simulink model "RF_FFT_Ex1"  (R2025a)
settings: Solver=ode45  StopTime=1024/10e3  EnableMultiTasking=on
InitFcn:
  | FFT_Size = 64;
undefined symbols (not defined in the file): i, S, vsva2488, xcvr1602
libraries: hdlBasic x15, dspsrcs4 x1, hdlDSPIP x1, dspxfrm3 x1, vmcUtilities x1
settings Model: Creator=dahlawat  LastModifiedBy=robg
settings SolverCC: AlgebraicLoopSolver=TrustRegion
settings DataIOCC: LimitDataPoints=on  SaveFormat=Array  ReturnWorkspaceOutputs=off
settings OptimizationCC: LifeSpan=inf
settings DebuggingCC: SolverPrmCheckMsg=warning  UnconnectedInputMsg=warning  UnconnectedOutputMsg=warning  UnconnectedLineMsg=warning  StateNameClashWarn=warning  SFUnexpectedBacktrackingDiag=warning  SFNoUnconditionalDefaultTransitionDiag=warning  SFExecutionAtInitializationDiag=none  ArithmeticOperatorsInVariantConditions=warning
settings HardwareCC: ProdBitPerPointer=32.0  ProdBitPerSizeT=32.0  ProdBitPerPtrDiffT=32.0  ProdLargestAtomicFloat=None  ProdIntDivRoundTo=Undefined  ProdEndianess=Unspecified  ProdWordSize=32.0  ProdHWDeviceType=32-bit Generic
settings ModelReferenceCC: EnableRefExpFcnMdlSchedulingChecks=on
settings SFSimCC: SimUseLocalCustomCode=off  CustomCodeUndefinedFunction=UseInterfaceOnly
settings RTWCC: RTWUseLocalCustomCode=off  GPUComputeCapability=3.5  DLArmComputeVersion=19.05
settings CodeAppCC: StateflowObjectComments=on
settings GRTTargetCC: TargetLangStandard=C89/C90 (ANSI)
settings ConfigComp: CovMetricSettings=dw  CovSaveCumulativeToWorkspaceVar=on  CovSaveSingleToWorkspaceVar=on  CovExternalEMLEnable=off

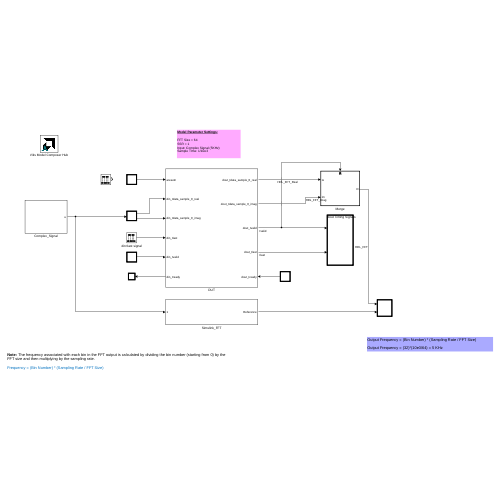
[thumbnail: Simulink's stored preview of the top-level diagram]
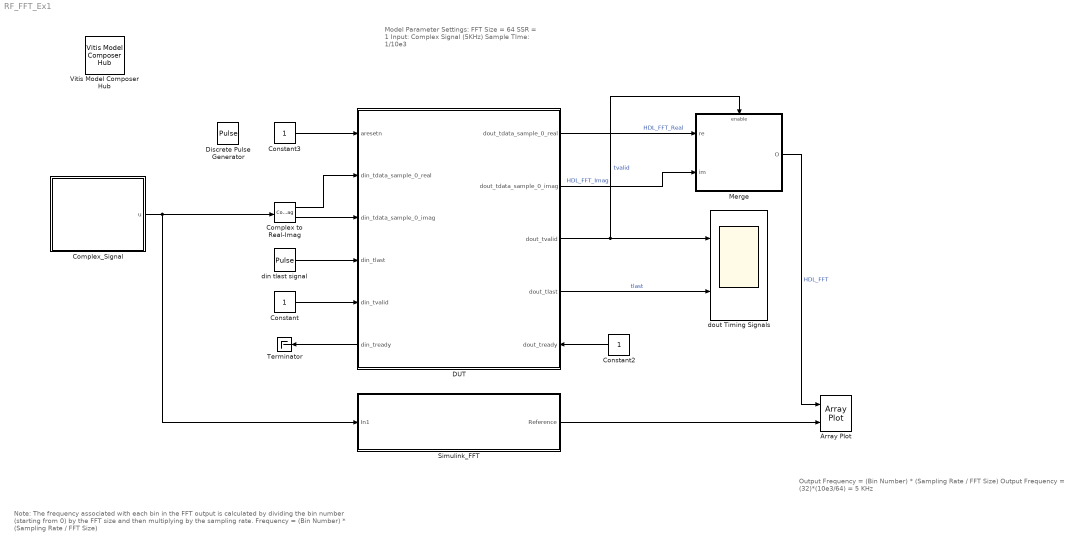
== system RF_FFT_Ex1 ==
  note: Output Frequency = (Bin Number) * (Sampling Rate / FFT Size)
      |
      | Output Frequency = (32)*(10e3/64) = 5 KHz
  note: Note: The frequency associated with each bin in the FFT output is calculated by dividing the bin number (starting from 0) by the FFT size and then multiplying by the sampling rate.
      |
      | Frequency = (Bin Number) * (Sampling Rate / FFT Size)
  note: Model Parameter Settings:
      |
      | FFT Size = 64
      | SSR = 1
      | Input: Complex Signal (5KHz)
      | Sample TIme: 1/10e3
  Array Plot : ArrayPlot  NumInputPorts=2  WindowPosition=[6.000000,33.000000,1920.000000,1149.000000,]  Visible=on  ScopeFrameLocation=window  YLimits=[-0.0625 0.5625]  ShowLegend=on
  Complex to Real-Imag : ComplexToRealImag
  Complex_Signal : Subsystem
  Constant : Constant
  Constant2 : Constant
  Constant3 : Constant
  DUT : Subsystem
      settings: PortSchema="{\"entries\":[{\"content\":{\"sides\":[{\"content\":{\"connectorIds\":[\"In1\",\"In2\",\"In3\",\"In4\",\"In5\",\"Out5\"]},\"type\":\"ConnectorPlacement.EquallySpacedRectSide\",\"uuid\":\"3c6f3837-184a-448e-85f8-bb0a441efaec\"},{\"content\":{\"connectorIds\":[\"Out1\",\"Out2\",\"Out3\",\"Out4\",\"In6\"],\"side\":\"RIGHT\"},\"type\":\"ConnectorPlacement.EquallySpacedRectSide\",\"uuid\":\"46fc4b89-da5b-4d62-9143-13f654c886da\"},{\"content\":{\"side\":\"TOP\"},\"type\":\"ConnectorPlacement.EquallySpacedRectSide\",\"uuid\":\"2ecc5b63-43c6-41c4-888c-4e2ddc41af1e\"}]},\"type\":\"ConnectorPlacement.EquallySpacedConnector\",\"uuid\":\"ba77804d-286f-47a8-b8da-0557eabd74b9\"}],\"packageUris\":[\"http://schema.mathworks.com/mf0/Connector/R2020b\"],\"version\":\"1.0\"}"
  Discrete Pulse Generator : DiscretePulseGenerator  Period=1  SampleTime=1/1e4
  Merge : Subsystem
  Simulink_FFT : Subsystem
  Terminator : Terminator
  Vitis Model Composer Hub : vmcUtilities/Vitis Model Composer Hub  Tag=genX  CodeGeneration=off  SubsystemName=DUT  CompilationType=HDLCompilation  SubsystemType=HDLNode  ExportTypeV2=IP Catalog  StartColumn=1  NumberOfColumns=1  TargetDirectory=./netlist  exportDesign=off  analyzeDesign=on  validateDesignOnHw=off  ExportType=HW Code  IpVendor=xilinx.com  IpLibrary=hls  IpVersion=1.0  IpHWLanguage=Verilog  AieCompilerOptions={}  AieSimulatorOptions={}  CreateTestbench=on  TestbenchStackSize=10  RunRtlSim=off  RunCSim=off  RunAieSim=on  enableSimulationTimeout=on  enableGraphIterations=on  AieSimTimeout=50000  AieGraphIterations=-1  RunAieSimProfiling=off  LaunchVitisAnalyzer=off  PlotOutput=off  RunX86Sim=off  X86SimTimeout=10  GenHwImage=off  GenLibadfXo=on  GenHwValidationCode=off  PlatformType=Not Specified  HwSystemType=Baremetal  HwValidationTarget=hw  ProjDevice=xcvr1602-vsva2488-2HP-i-S  ProjDevicePart=xcvr1602-vsva2488-2HP-i-S  AIEType=AIE  SamplePeriod=-1  ClockFrequency=200  DataPathParallelism=1  xilinxfamily=versalrf  part=xcvr1602  speed=-2HP-i-S  package=vsva2488  directory=./netlist/ip/DUT/src  testbench=off  incr_netlist=off  synthesis_tool=Vivado  clock_wrapper=Clock Enables  dbl_ovrd=According to Block Masks  dcm_input_clock_period=10  sysclk_period=10  simulink_period=1/1e4  eval_field=0  IPInfoJsonString="{\"DUTSubsystemName\":\"Vector_IFFT_FLOAT\",\"HDLSubsystem\":{\"SubsystemName\":\"Vector_IFFT_FLOAT\",\"IPName\":\"Vector_IFFT_FLOAT\",\"IPLibrary\":\"VMC\",\"IPVendor\":\"User Company\",\"IPVersion\":\"1.0\",\"TargetDirectory\":\"./netlist\",\"SubsystemDir\":\"./netlist/ip/Vector_IFFT_FLOAT\",\"FreqHz\":\"100000000\"},\"SubsystemTag\":\"HDLNode\"}"  LogFileName=/proj/xhdhdstaff5/sdegala/Head1/HEAD/2025_1_newBlocks/netlist/model_composer.log  NThreads=4  IPConfigFile=/tmp/vmctmp-sdegala/1167582/ipconfig.json
  din tlast signal : DiscretePulseGenerator  Period=FFT_Size  PhaseDelay=FFT_Size-1  SampleTime=1/1e4
  dout Timing Signals : Scope  NumInputPorts=2
      settings: ActiveDisplayYMinimum=-7.875  ActiveDisplayYMaximum=70.875
  wires:
  Complex to Real-Imag/1 -> DUT/2(din_tdata_sample_0_real)
  Complex to Real-Imag/2 -> DUT/3(din_tdata_sample_0_imag)
  DUT/3(dout_tvalid) -> dout Timing Signals/1, Merge/Enable  "tvalid"
  din tlast signal/1 -> DUT/4(din_tlast)
  DUT/1(dout_tdata_sample_0_real) -> Merge/1(re)  "HDL_FFT_Real"
  DUT/2(dout_tdata_sample_0_imag) -> Merge/2(im)  "HDL_FFT_Imag"
  Merge/1(O) -> Array Plot/1  "HDL_FFT"
  Complex_Signal/1(u) -> Simulink_FFT/1(In1), Complex to Real-Imag/1
  Simulink_FFT/1(Reference) -> Array Plot/2
  Constant/1 -> DUT/5(din_tvalid)
  Constant2/1 -> DUT/6(dout_tready)
  DUT/5(din_tready) -> Terminator/1
  Constant3/1 -> DUT/1(aresetn)
  DUT/4(dout_tlast) -> dout Timing Signals/2  "tlast"

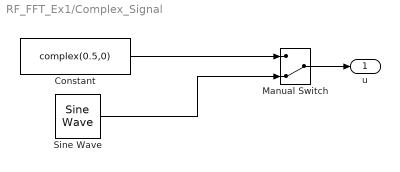
== system RF_FFT_Ex1/Complex_Signal ==
  Constant : Constant  Value=complex(0.5,0)  SampleTime=1/10e3
  Manual Switch : ManualSwitch  CurrentSetting=0
  Sine Wave : dspsrcs4/Sine Wave  Amplitude=0.5  Frequency=5e3  Phase=0  SampleMode=Discrete  OutComplex=Complex  CompMethod=Trigonometric fcn  TableSize=Speed  SampleTime=1/10e3  SamplesPerFrame=1  ResetState=Restart at time zero  OutputFrames=off  dataType=double  wordLen=16  udDataType=sfix(16)  fracBitsMode=Best precision  numFracBits=15  OutDataTypeStr=double  LastOutDataTypeStr=double
  u : Outport
  wires:
  Constant/1 -> Manual Switch/1
  Manual Switch/1 -> u/1
  Sine Wave/1 -> Manual Switch/2

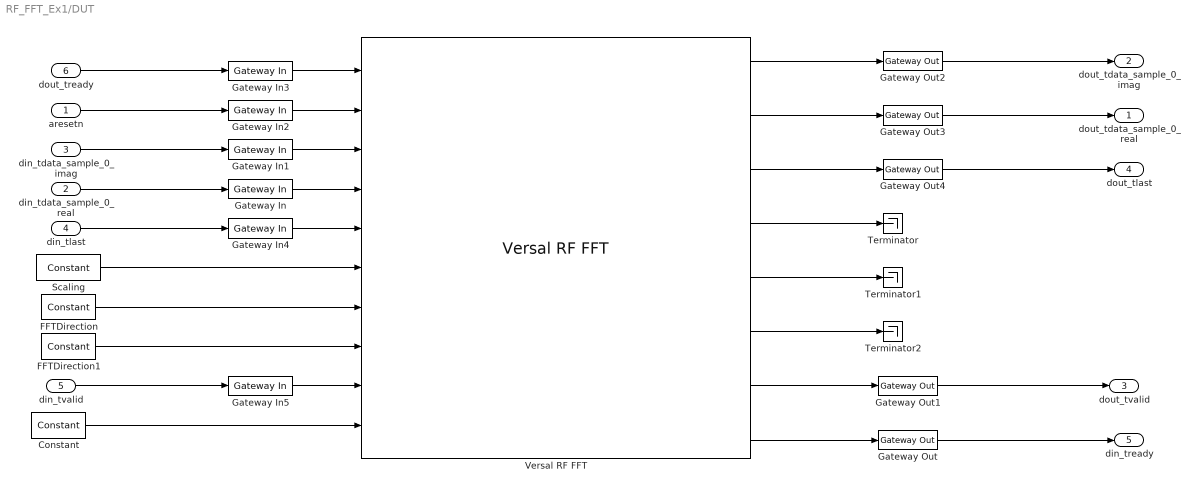
== system RF_FFT_Ex1/DUT ==
  aresetn : Inport
  din_tdata_sample_0_real : Inport  Port=2
  din_tdata_sample_0_imag : Inport  Port=3
  din_tlast : Inport  Port=4
  din_tvalid : Inport  Port=5
  dout_tready : Inport  Port=6
  Constant : hdlBasic/Constant  const=1.0  gui_display_data_type=Boolean  arith_type=Boolean  n_bits=16  bin_pt=14  preci_type=Single  exp_width=8  frac_width=24  explicit_period=on  period=1/1e4  XmcBlockStatus=1  maskContainerNames=tabcontainer1  block_type=constant  block_config=sysgen:Constant_config
  FFTDirection : hdlBasic/Constant  const=1.0  gui_display_data_type=Fixed-point  arith_type=Unsigned  n_bits=1  bin_pt=0  preci_type=Single  exp_width=8  frac_width=24  explicit_period=on  period=1/1e4  XmcBlockStatus=1  maskContainerNames=tabcontainer1  block_type=constant  block_config=sysgen:Constant_config
  FFTDirection1 : hdlBasic/Constant  const=log2(FFT_Size)  gui_display_data_type=Fixed-point  arith_type=Unsigned  n_bits=4  bin_pt=0  preci_type=Single  exp_width=8  frac_width=24  explicit_period=on  period=1/1e4  XmcBlockStatus=1  maskContainerNames=tabcontainer1  block_type=constant  block_config=sysgen:Constant_config
  Gateway In : hdlBasic/Gateway In  gui_display_data_type=Fixed-point  arith_type=Signed (2's comp)  n_bits=18  bin_pt=17  preci_type=Single  exp_width=8  frac_width=24  rows=1  columns=1  quantization="Round  (unbiased: +/- Inf)"  overflow=Saturate  period=1/1e4  UseAsADC=off  ADCChannel='1'  interface=None  automatic_assignment=on  address_offset=hex2dec('00')  intf_name=''  intf_description=''  default_value=0  timing_constraint=None  locs_specified=off  LOCs={}  io_standard={}  inherit_from_input=off  hdl_port=on  XmcBlockStatus=1  maskContainerNames=group4  block_type=gatewayin  block_config=sysgen:gateway_in_config  block_width_w=590  block_height_w=620  block_width=640  block_height=850
  Gateway In1 : hdlBasic/Gateway In  gui_display_data_type=Fixed-point  arith_type=Signed (2's comp)  n_bits=18  bin_pt=17  preci_type=Single  exp_width=8  frac_width=24  rows=1  columns=1  quantization="Round  (unbiased: +/- Inf)"  overflow=Saturate  period=1/1e4  UseAsADC=off  ADCChannel='1'  interface=None  automatic_assignment=on  address_offset=hex2dec('00')  intf_name=''  intf_description=''  default_value=0  timing_constraint=None  locs_specified=off  LOCs={}  io_standard={}  inherit_from_input=off  hdl_port=on  XmcBlockStatus=1  maskContainerNames=group4  block_type=gatewayin  block_config=sysgen:gateway_in_config  block_width_w=590  block_height_w=620  block_width=640  block_height=850
  Gateway In{2..5} (4 alike) : hdlBasic/Gateway In  gui_display_data_type=Boolean  arith_type=Boolean  n_bits=16  bin_pt=14  preci_type=Single  exp_width=8  frac_width=24  rows=1  columns=1  quantization="Round  (unbiased: +/- Inf)"  overflow=Saturate  period=1/1e4  UseAsADC=off  ADCChannel='1'  interface=None  automatic_assignment=on  address_offset=hex2dec('00')  intf_name=''  intf_description=''  default_value=0  timing_constraint=None  locs_specified=off  LOCs={}  io_standard={}  inherit_from_input=off  hdl_port=on  XmcBlockStatus=1  maskContainerNames=group4  block_type=gatewayin  block_config=sysgen:gateway_in_config  block_width_w=590  block_height_w=620  block_width=640  block_height=850
  Gateway Out : hdlBasic/Gateway Out  inherit_from_input=off  bool_to_boolean=off  hdl_port=on  rows=1  columns=1  UseAsDAC=off  DACChannel='1'  interface=None  automatic_assignment=on  address_offset=hex2dec('00')  intf_name=''  intf_description=''  timing_constraint=None  locs_specified=off  LOCs={}  io_standard={}  XmcBlockStatus=1  maskContainerNames=group4  block_type=gatewayout  block_config=sysgen:gateway_out_config  block_width_w=590  block_height_w=620  block_width=620  block_height=750
  Gateway Out1 : hdlBasic/Gateway Out  inherit_from_input=on  bool_to_boolean=off  hdl_port=on  rows=1  columns=1  UseAsDAC=off  DACChannel='1'  interface=None  automatic_assignment=on  address_offset=hex2dec('00')  intf_name=''  intf_description=''  timing_constraint=None  locs_specified=off  LOCs={}  io_standard={}  XmcBlockStatus=1  maskContainerNames=group4  block_type=gatewayout  block_config=sysgen:gateway_out_config  block_width_w=590  block_height_w=620  block_width=620  block_height=750
  Gateway Out2 : hdlBasic/Gateway Out  inherit_from_input=off  bool_to_boolean=off  hdl_port=on  rows=1  columns=1  UseAsDAC=off  DACChannel='1'  interface=None  automatic_assignment=on  address_offset=hex2dec('00')  intf_name=''  intf_description=''  timing_constraint=None  locs_specified=off  LOCs={}  io_standard={}  XmcBlockStatus=1  maskContainerNames=group4  block_type=gatewayout  block_config=sysgen:gateway_out_config  block_width_w=590  block_height_w=620  block_width=620  block_height=750
  Gateway Out3 : hdlBasic/Gateway Out  inherit_from_input=off  bool_to_boolean=off  hdl_port=on  rows=1  columns=1  UseAsDAC=off  DACChannel='1'  interface=None  automatic_assignment=on  address_offset=hex2dec('00')  intf_name=''  intf_description=''  timing_constraint=None  locs_specified=off  LOCs={}  io_standard={}  XmcBlockStatus=1  maskContainerNames=group4  block_type=gatewayout  block_config=sysgen:gateway_out_config  block_width_w=590  block_height_w=620  block_width=620  block_height=750
  Gateway Out4 : hdlBasic/Gateway Out  inherit_from_input=on  bool_to_boolean=off  hdl_port=on  rows=1  columns=1  UseAsDAC=off  DACChannel='1'  interface=None  automatic_assignment=on  address_offset=hex2dec('00')  intf_name=''  intf_description=''  timing_constraint=None  locs_specified=off  LOCs={}  io_standard={}  XmcBlockStatus=1  maskContainerNames=group4  block_type=gatewayout  block_config=sysgen:gateway_out_config  block_width_w=590  block_height_w=620  block_width=620  block_height=750
  Scaling : hdlBasic/Constant  const=1/FFT_Size  gui_display_data_type=Fixed-point  arith_type=Unsigned  n_bits=13  bin_pt=13  preci_type=Single  exp_width=8  frac_width=24  explicit_period=on  period=1/1e4  XmcBlockStatus=1  maskContainerNames=tabcontainer1  block_type=constant  block_config=sysgen:Constant_config
  Terminator : Terminator
  Terminator1 : Terminator
  Terminator2 : Terminator
  Versal RF FFT : hdlDSPIP/Versal RF FFT  sample_rate=1  fft_max_point_size_temp=64  fft_max_point_size=6  fft_scaling=on  fft_reorder=on  data_width_in=18  data_width_out=18  events=off  ip_name=Versal RF FFT  enable_all_ports=false  mode=Streaming FFT  ip_version=1.2  dsptool_ready=false  ipcore_usecache=true  ipcore_useipmodelcache=true  wrapper_available=true  port_translation_map={ 'S_AXIS_aclken' => 'en', 'aresetn' => 'rst' }  structural_sim=true  ipcore_do_not_force_period=true  XmcBlockStatus=1  maskContainerNames=tabcontainer1  block_type=vrf_fft_v1_0  block_config=sysgen:rodinimport_config  simulation_type=xsim
  dout_tdata_sample_0_real : Outport
  dout_tdata_sample_0_imag : Outport  Port=2
  dout_tvalid : Outport  Port=3
  dout_tlast : Outport  Port=4
  din_tready : Outport  Port=5
  wires:
  din_tdata_sample_0_real/1 -> Gateway In/1
  Versal RF FFT/7 -> Gateway Out1/1
  Gateway Out1/1 -> dout_tvalid/1
  din_tdata_sample_0_imag/1 -> Gateway In1/1
  Gateway In1/1 -> Versal RF FFT/3
  Gateway In/1 -> Versal RF FFT/4
  aresetn/1 -> Gateway In2/1
  Constant/1 -> Versal RF FFT/10
  FFTDirection1/1 -> Versal RF FFT/8
  Versal RF FFT/8 -> Gateway Out/1
  Versal RF FFT/6 -> Terminator2/1
  Versal RF FFT/5 -> Terminator1/1
  Versal RF FFT/4 -> Terminator/1
  Versal RF FFT/3 -> Gateway Out4/1
  Versal RF FFT/2 -> Gateway Out3/1
  Versal RF FFT/1 -> Gateway Out2/1
  Gateway Out2/1 -> dout_tdata_sample_0_imag/1
  Gateway Out3/1 -> dout_tdata_sample_0_real/1
  Gateway Out4/1 -> dout_tlast/1
  Gateway Out/1 -> din_tready/1
  FFTDirection/1 -> Versal RF FFT/7
  Gateway In4/1 -> Versal RF FFT/5
  din_tlast/1 -> Gateway In4/1
  Gateway In2/1 -> Versal RF FFT/2
  Scaling/1 -> Versal RF FFT/6
  Gateway In5/1 -> Versal RF FFT/9
  din_tvalid/1 -> Gateway In5/1
  Gateway In3/1 -> Versal RF FFT/1
  dout_tready/1 -> Gateway In3/1

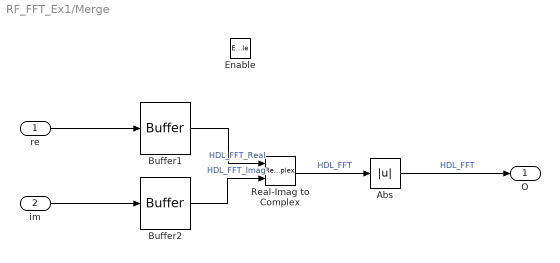
== system RF_FFT_Ex1/Merge ==
  re : Inport
  im : Inport  Port=2
  Enable : EnablePort
  Abs : Abs  SaturateOnIntegerOverflow=off
  Buffer1 : Buffer  OutputFrames=off
  Buffer2 : Buffer  OutputFrames=off
  Real-Imag to Complex : RealImagToComplex
  O : Outport
  wires:
  Real-Imag to Complex/1 -> Abs/1  "HDL_FFT"
  Buffer2/1 -> Real-Imag to Complex/2  "HDL_FFT_Imag"
  im/1 -> Buffer2/1
  Buffer1/1 -> Real-Imag to Complex/1  "HDL_FFT_Real"
  re/1 -> Buffer1/1
  Abs/1 -> O/1  "HDL_FFT"

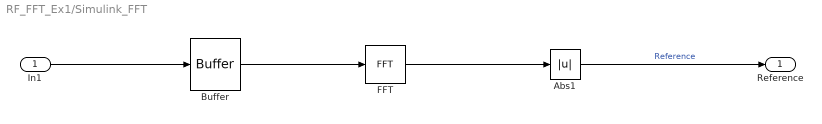
== system RF_FFT_Ex1/Simulink_FFT ==
  In1 : Inport
  Abs1 : Abs  SaturateOnIntegerOverflow=off
  Buffer : Buffer  OutputFrames=off
  FFT : dspxfrm3/FFT  FFTImplementation=Auto  CompMethod=Table lookup  TableOpt=NEW  TableOptActive=Speed  BitRevOrder=off  Normalize=on  InheritFFTLength=on  FFTLength=64  WrapInput=on  roundingMode=Floor  overflowMode=off  firstCoeffDataTypeStr=Inherit: Same word length as input  firstCoeffLastDataTypeStr=Inherit: Same word length as input  outputMin=[]  outputMax=[]
  Reference : Outport
  wires:
  FFT/1 -> Abs1/1
  Abs1/1 -> Reference/1  "Reference"
  Buffer/1 -> FFT/1
  In1/1 -> Buffer/1
